simulink subsystem "Extended_Model"  (R2022b)
settings: Solver=VariableStepAuto  StartTime=0.0  StopTime=10.0  RelTol=1e-3
model mask{motor_model=0}
  mask prompts: motor_model "Motor Parameter struct:"
undefined symbols (not defined in the file): motor
settings Model: Creator=gotta  LastModifiedBy=gotta

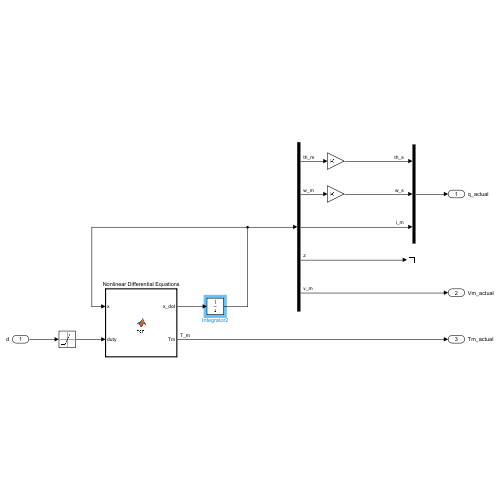
[thumbnail: Simulink's stored preview of the top-level diagram]
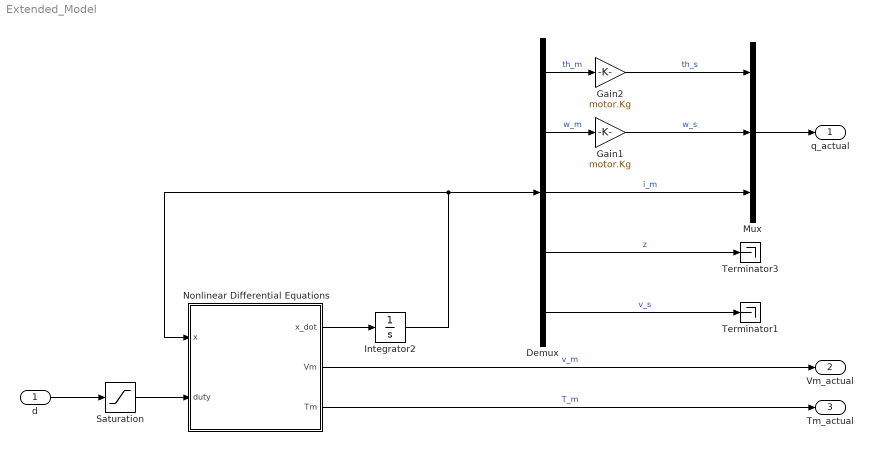
== system Extended_Model ==
  d : Inport
  Demux : Demux  Outputs=5
  Gain1 : Gain  Gain=motor.Kg
  Gain2 : Gain  Gain=motor.Kg
  Integrator2 : Integrator  InitialCondition=zeros(5, 1)
  Mux : Mux  Inputs=3
  Nonlinear Differential Equations : MATLAB Function  TreatAsAtomicUnit=on
  Saturation : Saturate  UpperLimit=1  LowerLimit=-1
  Terminator1 : Terminator
  Terminator3 : Terminator
  q_actual : Outport
  Vm_actual : Outport  Port=2
  Tm_actual : Outport  Port=3
  wires:
  Demux/1 -> Gain2/1  "th_m"
  Demux/3 -> Mux/3  "i_m"
  Nonlinear Differential Equations/3(Tm) -> Tm_actual/1  "T_m"
  Demux/2 -> Gain1/1  "w_m"
  d/1 -> Saturation/1
  Gain1/1 -> Mux/2  "w_s"
  Mux/1 -> q_actual/1
  Demux/4 -> Terminator3/1  "z"
  Integrator2/1 -> Nonlinear Differential Equations/1(x), Demux/1
  Saturation/1 -> Nonlinear Differential Equations/2(duty)
  Nonlinear Differential Equations/1(x_dot) -> Integrator2/1
  Gain2/1 -> Mux/1  "th_s"
  Nonlinear Differential Equations/2(Vm) -> Vm_actual/1  "v_m"
  Demux/5 -> Terminator1/1  "v_s"

== matlab function Extended_Model/Nonlinear Differential Equations ==
  data: x input; duty input; x_dot output; Vm output; motor_model parameter; Tm output
function [x_dot, Vm, Tm] = fcn(x, duty, motor_model)

% State vector unpacking
w_m = x(2);
z = x(4);
v_s = x(5);

% Additional parameters
Cs = 100e-9;    % sensor filter capacitor   [F]
Rs = 0.01;      % sensor shunt resistor     [Ohm]


% F and G matrices parameters
f22 = -(motor_model.Be + motor_model.s1) / motor_model.Je;
f23 = motor_model.Kphi / motor_model.Je;
f24 = -motor_model.s0 / motor_model.Je;

f32 = -motor_model.Kphi / motor_model.La;
f33 = -motor_model.Ra / motor_model.La;
f35 = -1/motor_model.La;

f53 = 2/Cs;
f55 = -1/(Cs*Rs);


g3 = motor_model.Vcc/motor_model.La;


% F and G matrices
F = [
    0, 1,   0,   0,   0;
    0, f22, f23, f24, 0;
    0, f32, f33, 0,   f35;
    0, 1,   0,   0,   0; 
    0, 0,   f53, 0,   f55; 
    ];

G = [0; 0; g3; 0; 0];


% Stribeck curve
Tf = motor_model.Tc + (motor_model.Tsb - motor_model.Tc)*exp(-(w_m / motor_model.w_sb)^2);

% LuGre function
Zl = motor_model.s0*abs(w_m)*z / Tf;


% W matrix
W = [0; motor_model.s1*Zl / motor_model.Je; 0; -Zl; 0];


% Outputs
x_dot = F*x + G*duty + W;
Vm = motor_model.Vcc*duty - v_s;
Tm = motor_model.s0*z + motor_model.s1*(w_m - Zl) + motor_model.Be*w_m;
